simulink model "part2_1"  (R2017b)
settings: Solver=VariableStepAuto  StartTime=0.0  StopTime=2  RelTol=1e-3
settings Model: Creator=Li  LastModifiedBy=think

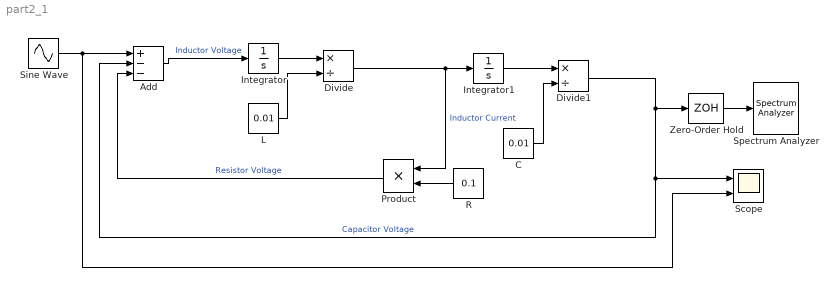
== system part2_1 ==
  Add : Sum  Inputs=+--
  C : Constant  Value=0.01
  Divide : Product  Inputs=*/
  Divide1 : Product  Inputs=*/
  Integrator : Integrator
  Integrator1 : Integrator
  L : Constant  Value=0.01
  Product : Product
  R : Constant  Value=0.1
  Scope : Scope  NumInputPorts=2
  Sine Wave : Sin  Frequency=100*5  SampleTime=0
  Spectrum Analyzer : SpectrumAnalyzer
  Zero-Order Hold : ZeroOrderHold  SampleTime=2^(-10)
  wires:
  Integrator/1 -> Divide/1
  L/1 -> Divide/2
  Divide/1 -> Integrator1/1, Product/1  "Inductor Current"
  Integrator1/1 -> Divide1/1
  R/1 -> Product/2
  Add/1 -> Integrator/1  "Inductor Voltage"
  Product/1 -> Add/3  "Resistor Voltage"
  Divide1/1 -> Zero-Order Hold/1, Add/2, Scope/1  "Capacitor Voltage"
  C/1 -> Divide1/2
  Zero-Order Hold/1 -> Spectrum Analyzer/1
  Sine Wave/1 -> Scope/2, Add/1
